simulink model "Decision_Module"  (R2015a)
settings: Solver=FixedStepDiscrete  StartTime=0.0  StopTime=10.0  FixedStep=delta_t  RelTol=1e-3
undefined symbols (not defined in the file): D, delta_t, I, Kd, Kp, M_tilde, psi_dot_max, psi_max, S, S_pinv
settings Model: Creator=Kerianne  LastModifiedBy=Kerianne
settings DataIOCC: SaveFormat=Structure
settings OptimizationCC: InlineParams=on  ExpressionDepthLimit=2147483647
settings DebuggingCC: UnderspecifiedInitializationDetection=Classic  MergeDetectMultiDrivingBlocksExec=none  SolverPrmCheckMsg=warning  StateNameClashWarn=warning

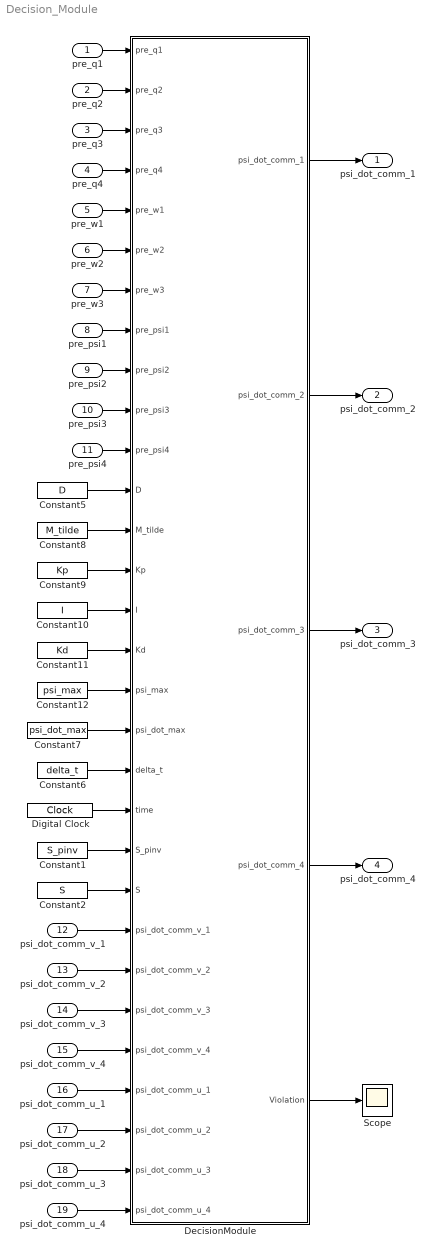
== system Decision_Module ==
  pre_q1 : Inport
  pre_q2 : Inport  Port=2
  pre_q3 : Inport  Port=3
  pre_q4 : Inport  Port=4
  pre_w1 : Inport  Port=5
  pre_w2 : Inport  Port=6
  pre_w3 : Inport  Port=7
  pre_psi1 : Inport  Port=8
  pre_psi2 : Inport  Port=9
  pre_psi3 : Inport  Port=10
  pre_psi4 : Inport  Port=11
  psi_dot_comm_v_1 : Inport  Port=12
  psi_dot_comm_v_2 : Inport  Port=13
  psi_dot_comm_v_3 : Inport  Port=14
  psi_dot_comm_v_4 : Inport  Port=15
  psi_dot_comm_u_1 : Inport  Port=16
  psi_dot_comm_u_2 : Inport  Port=17
  psi_dot_comm_u_3 : Inport  Port=18
  psi_dot_comm_u_4 : Inport  Port=19
  Constant1 : Constant  Value=S_pinv
  Constant10 : Constant  Value=I
  Constant11 : Constant  Value=Kd
  Constant12 : Constant  Value=psi_max
  Constant2 : Constant  Value=S
  Constant5 : Constant  Value=D
  Constant6 : Constant  Value=delta_t
  Constant7 : Constant  Value=psi_dot_max
  Constant8 : Constant  Value=M_tilde
  Constant9 : Constant  Value=Kp
  DecisionModule : MATLAB Function  TreatAsAtomicUnit=on
  Digital Clock : DigitalClock  SampleTime=delta_t
  Scope : Scope
  psi_dot_comm_1 : Outport
  psi_dot_comm_2 : Outport  Port=2
  psi_dot_comm_3 : Outport  Port=3
  psi_dot_comm_4 : Outport  Port=4
  wires:
  Constant6/1 -> DecisionModule/19(delta_t)
  Constant7/1 -> DecisionModule/18(psi_dot_max)
  Constant12/1 -> DecisionModule/17(psi_max)
  Constant11/1 -> DecisionModule/16(Kd)
  Constant10/1 -> DecisionModule/15(I)
  Constant9/1 -> DecisionModule/14(Kp)
  Constant8/1 -> DecisionModule/13(M_tilde)
  Constant5/1 -> DecisionModule/12(D)
  pre_psi3/1 -> DecisionModule/10(pre_psi3)
  pre_psi2/1 -> DecisionModule/9(pre_psi2)
  pre_psi1/1 -> DecisionModule/8(pre_psi1)
  pre_w3/1 -> DecisionModule/7(pre_w3)
  pre_w2/1 -> DecisionModule/6(pre_w2)
  pre_w1/1 -> DecisionModule/5(pre_w1)
  pre_q4/1 -> DecisionModule/4(pre_q4)
  pre_q3/1 -> DecisionModule/3(pre_q3)
  pre_q2/1 -> DecisionModule/2(pre_q2)
  pre_q1/1 -> DecisionModule/1(pre_q1)
  DecisionModule/3(psi_dot_comm_3) -> psi_dot_comm_3/1
  DecisionModule/1(psi_dot_comm_1) -> psi_dot_comm_1/1
  DecisionModule/2(psi_dot_comm_2) -> psi_dot_comm_2/1
  Constant1/1 -> DecisionModule/21(S_pinv)
  DecisionModule/4(psi_dot_comm_4) -> psi_dot_comm_4/1
  pre_psi4/1 -> DecisionModule/11(pre_psi4)
  Constant2/1 -> DecisionModule/22(S)
  psi_dot_comm_v_1/1 -> DecisionModule/23(psi_dot_comm_v_1)
  psi_dot_comm_v_2/1 -> DecisionModule/24(psi_dot_comm_v_2)
  psi_dot_comm_v_3/1 -> DecisionModule/25(psi_dot_comm_v_3)
  psi_dot_comm_v_4/1 -> DecisionModule/26(psi_dot_comm_v_4)
  psi_dot_comm_u_1/1 -> DecisionModule/27(psi_dot_comm_u_1)
  psi_dot_comm_u_2/1 -> DecisionModule/28(psi_dot_comm_u_2)
  psi_dot_comm_u_3/1 -> DecisionModule/29(psi_dot_comm_u_3)
  psi_dot_comm_u_4/1 -> DecisionModule/30(psi_dot_comm_u_4)
  Digital Clock/1 -> DecisionModule/20(time)
  DecisionModule/5(Violation) -> Scope/1

== matlab function Decision_Module/DecisionModule ==
  data: pre_q1 input; pre_q2 input; pre_q3 input; pre_q4 input; pre_w1 input; pre_w2 input; pre_w3 input; pre_psi1 input; pre_psi2 input; pre_psi3 input; pre_psi4 input; psi_dot_comm_1 output; D input; M_tilde input; Kp input; I input; Kd input; psi_max input; psi_dot_max input; delta_t input; time input; psi_dot_comm_2 output; psi_dot_comm_3 output; psi_dot_comm_4 output; S_pinv input; S input; psi_dot_comm_v_1 input; psi_dot_comm_v_2 input; psi_dot_comm_v_3 input; psi_dot_comm_v_4 input; psi_dot_comm_u_1 input; psi_dot_comm_u_2 input; psi_dot_comm_u_3 input; psi_dot_comm_u_4 input; Violation output
function [psi_dot_comm_1, psi_dot_comm_2, psi_dot_comm_3,psi_dot_comm_4,Violation] = fcn(pre_q1,pre_q2,pre_q3,pre_q4,pre_w1,pre_w2,pre_w3,pre_psi1,pre_psi2,pre_psi3,pre_psi4,D,M_tilde,Kp,I,Kd,psi_max,psi_dot_max,delta_t,time,S_pinv,S,psi_dot_comm_v_1,psi_dot_comm_v_2,psi_dot_comm_v_3,psi_dot_comm_v_4,psi_dot_comm_u_1,psi_dot_comm_u_2,psi_dot_comm_u_3,psi_dot_comm_u_4)
% Decision Module for Reaction Wheel Control
% Author: Kerianne Gross, AFRL/RQQA, kerianne.gross@us.af.mil
% Last Updated: 
% 20 November 2015 
% 
% Note: This version of the Decision Module does not keep a history of
% whether the unverified controller has previously violated the safety
% properties. So if the unverified control sends a signal that no longer
% violates the properties, the Decision Module will switch back. In many
% cases this is not desireable. In general, if the unverified controller
% violates the safety properties, it cannot be trusted unless an action
% such as a reset or redesign is implemented. In some cases, however, an
% RTA system may be designed to switch control back and forth between the
% unverified and verified controller depending on whether the system is in
% the operating region of the unverified controller.
%
% This is a decision module that takes in the current state of the
% spacecraft, the outputs of the verified PID controller, and the outputs
% of the unverified blackbox controller and determines which controller
% signals make it out.
% 1) Check to see if unverified commanded acceleration (psi_dot_comm_u_x)
%    is > than max commanded acceleration (psi_dot_max) for any of the 
%    wheels. IF acceleration boundary is VIOLATED (psi_dot_comm_u_x > 
%    psi_dot_max),then use verified commanded acceleration signal  
%    (psi_dot_comm_v_x) for all wheels. 
% 2) Check to see if unverified commanded acceleration (psi_dot_comm_u_x)
%    would cause the wheel velocity (psi(x) to exceend the max velocity 
%    (psi_max) for any of the wheels. IF acceleration boundary is VIOLATED,
%    then use verified commanded acceleration signal (psi_dot_comm_v_x) for 
%    all wheels.
% 3) If none of the above conditions are violated, use the unverified
%    signal
% 
% DISCUSSION
%  > Why not just switch out the 1 bad signal, rather than all of the 
%    signals? Well, if one signal is 
%    bad, the unverified controller is no longer considered trustworthy 
%    until all signals are in bounds again. Depending on the criticality of 
%    the signal, one may want to add a flag to show that a violation 
%    occurred and use a different switching mechanism to switch back.
%  > There may be other characteristics you are trying to protect against
%    too, for instance, maybe you don't wan the spacecraft angular velocity
%    (w) to exceed a threshold, because it would make it very difficult to
%    recover beyond that threshold. These conditions just need to be listed
%    in order of precedence.


     % States at the end fot he last time step
    q       = [pre_q1,pre_q2,pre_q3,pre_q4];    %s/c quaternion
    omega   = [pre_w1,pre_w2,pre_w3];           %s/c angular rates 
    psi     = [pre_psi1,pre_psi2,pre_psi3,pre_psi4];     %RWA angle rates
        
    % Checks done in order of precedence from top to bottom
%    persistent Violation
%    if isempty(Violation)
%        Violation = 0;
%        Violation_flag = 0;
%    end
    if (abs(psi_dot_comm_u_1) >= psi_dot_max || ...
        abs(psi_dot_comm_u_2) >= psi_dot_max || ...
        abs(psi_dot_comm_u_3) >= psi_dot_max || ...
        abs(psi_dot_comm_u_4) >= psi_dot_max || ...
        abs(psi(1)+ psi_dot_comm_u_1*delta_t) >= psi_max || ...
        abs(psi(2)+ psi_dot_comm_u_2*delta_t) >= psi_max || ...
        abs(psi(3)+ psi_dot_comm_u_3*delta_t) >= psi_max || ...
        abs(psi(4)+ psi_dot_comm_u_4*delta_t) >= psi_max)
        psi_dot_comm_1 = psi_dot_comm_v_1;
        psi_dot_comm_2 = psi_dot_comm_v_2;
        psi_dot_comm_3 = psi_dot_comm_v_3;
        psi_dot_comm_4 = psi_dot_comm_v_4;
        
        Violation = 1;
    else 
        
        psi_dot_comm_1 = psi_dot_comm_u_1;
        psi_dot_comm_2 = psi_dot_comm_u_2;
        psi_dot_comm_3 = psi_dot_comm_u_3;
        psi_dot_comm_4 = psi_dot_comm_u_4;
        Violation = 0;
    end
    

%     % CHECK 1: PREVIOUSLY VIOLATED
%     if (Violation == 1)
%         psi_dot_comm_1 = psi_dot_comm_v_1;
%         psi_dot_comm_2 = psi_dot_comm_v_2;
%         psi_dot_comm_3 = psi_dot_comm_v_3;
%         psi_dot_comm_4 = psi_dot_comm_v_4; 
%         Violation_flag = 1;
%     % CHECK 2: VIOLATION OF RW MAX ANGULAR ACCELERATION (PSI_DOT_MAX)
%     elseif  abs(psi_dot_comm_u_1) >= psi_dot_max || abs(psi_dot_comm_u_2) >= ...
%             psi_dot_max || abs(psi_dot_comm_u_3) >= psi_dot_max || ...
%             abs(psi_dot_comm_u_4) >= psi_dot_max
%         psi_dot_comm_1 = psi_dot_comm_v_1;
%         psi_dot_comm_2 = psi_dot_comm_v_2;
%         psi_dot_comm_3 = psi_dot_comm_v_3;
%         psi_dot_comm_4 = psi_dot_comm_v_4;
%         % Outputs for debugging - not compatible with SLDV
%         % fprintf('Acceleration Violation');
%         % time
%         Violation_flag = 1;
%     % CHECK 3: VIOLATION OF RW MAX ANGULAR VELOCITY (PSI_MAX)
%     elseif abs(psi(1)+ psi_dot_comm_u_1*delta_t) >= psi_max || ...
%            abs(psi(2)+ psi_dot_comm_u_2*delta_t) >= psi_max || ...
%            abs(psi(3)+ psi_dot_comm_u_3*delta_t) >= psi_max || ...
%            abs(psi(4)+ psi_dot_comm_u_4*delta_t) >= psi_max
%         psi_dot_comm_1 = psi_dot_comm_v_1;
%         psi_dot_comm_2 = psi_dot_comm_v_2;
%         psi_dot_comm_3 = psi_dot_comm_v_3;
%         psi_dot_comm_4 = psi_dot_comm_v_4;
%         % Outputs for debugging - not compatible with SLDV
%         %fprintf('Velocity Violation');
%         %time
%         Violation_flag = 1;
%     % NO VIOLATIONS EXIST
%     elseif Violation == 0
%         psi_dot_comm_1 = psi_dot_comm_u_1;
%         psi_dot_comm_2 = psi_dot_comm_u_2;
%         psi_dot_comm_3 = psi_dot_comm_u_3;
%         psi_dot_comm_4 = psi_dot_comm_u_4;
%         Violation_flag = 0;     
%     % ERROR CASE : LOGIC PROBLEM
%     else
%         %fprintf('Error');
%         psi_dot_comm_1 = psi_dot_comm_v_1;
%         psi_dot_comm_2 = psi_dot_comm_v_2;
%         psi_dot_comm_3 = psi_dot_comm_v_3;
%         psi_dot_comm_4 = psi_dot_comm_v_4;
%         Violation_flag = 0;        
%     end

%Violation = Violation_flag;
